simulink subsystem "OrbitPropSubSys"  (R2022b)
settings: Solver=VariableStepAuto  StartTime=0.0  StopTime=10.0  RelTol=1e-3
settings Model: Creator=BlueR  LastModifiedBy=BlueR

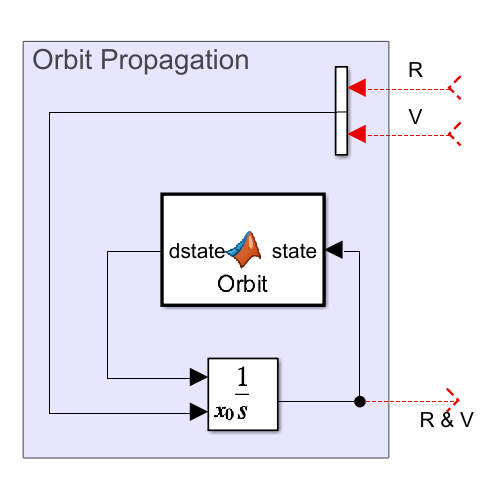
[thumbnail: Simulink's stored preview of the top-level diagram]
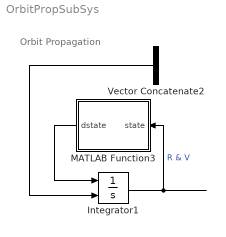
== system OrbitPropSubSys ==
  note: Orbit Propagation
  Integrator1 : Integrator  InitialConditionSource=external  ContinuousStateAttributes='orbit'
  MATLAB Function3 : MATLAB Function  TreatAsAtomicUnit=on
  Vector Concatenate2 : Concatenate
  wires:
  MATLAB Function3/1(dstate) -> Integrator1/1
  Vector Concatenate2/1 -> Integrator1/2
  Integrator1/1 -> MATLAB Function3/1(state)  "R & V"
  ? -> Vector Concatenate2/1  "R"
  ? -> Vector Concatenate2/2  "V"

== matlab function OrbitPropSubSys/MATLAB Function3 ==
  data: state input; dstate output
function dstate  = Orbit(state)

muearth = 398600;
x = state(1);
y = state(2);
z = state(3);
dx = state(4);
dy = state(5);
dz = state(6);
r = norm([x y z]);
ddx = -muearth*x/r^3;
ddy = -muearth*y/r^3;
ddz = -muearth*z/r^3;
dR = [dx; dy; dz];
dV = [ddx; ddy; ddz];

dstate = [dR;dV];

end
